simulink model "HevP4ReferenceApplication"  (R2020a)
settings: Solver=ode23tb  StartTime=0  StopTime=1800  RelTol=1e-3  EnableMultiTasking=on
undefined symbols (not defined in the file): sigbuilder_block
libraries: autolibshared x2
(part 2 of 2)

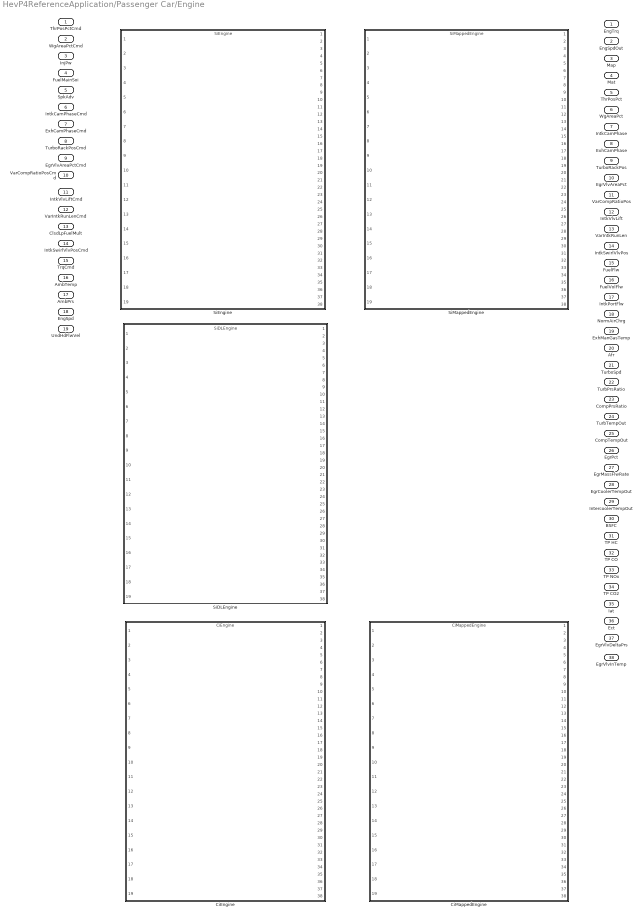
== system HevP4ReferenceApplication/Passenger Car/Engine ==
  ThrPosPctCmd : Inport
  WgAreaPctCmd : Inport  Port=2
  InjPw : Inport  Port=3
  FuelMainSoi : Inport  Port=4
  SpkAdv : Inport  Port=5
  IntkCamPhaseCmd : Inport  Port=6
  ExhCamPhaseCmd : Inport  Port=7
  TurboRackPosCmd : Inport  Port=8
  EgrVlvAreaPctCmd : Inport  Port=9
  VarCompRatioPosCmd : Inport  Port=10
  IntkVlvLiftCmd : Inport  Port=11
  VarIntkRunLenCmd : Inport  Port=12
  ClsdLpFuelMult : Inport  Port=13
  IntkSwirlVlvPosCmd : Inport  Port=14
  TrqCmd : Inport  Port=15
  AmbTemp : Inport  Port=16
  AmbPrs : Inport  Port=17
  EngSpd : Inport  Port=18
  UndHdFlwVel : Inport  Port=19
  CiEngine : ModelReference  ModelNameDialog=CiEngine.slx  SimulationMode=Normal  VariantControl=CiEngine  ModelReferenceVersion=1.370
  CiMappedEngine : ModelReference  ModelNameDialog=CiMappedEngine.slx  SimulationMode=Normal  VariantControl=CiMappedEngine  ModelReferenceVersion=1.321
  SiDLEngine : ModelReference  ModelNameDialog=SiDLEngine  SimulationMode=Normal  VariantControl=SiDLEngine  ModelReferenceVersion=1.459
  SiEngine : ModelReference  ModelNameDialog=SiEngine.slx  SimulationMode=Normal  VariantControl=SiEngine  ModelReferenceVersion=1.573
  SiMappedEngine : ModelReference  ModelNameDialog=SiMappedEngine.slx  SimulationMode=Normal  VariantControl=SiMappedEngine  ModelReferenceVersion=1.331
  EngTrq : Outport  VectorParamsAs1DForOutWhenUnconnected=off
  EngSpdOut : Outport  Port=2  VectorParamsAs1DForOutWhenUnconnected=off
  Map : Outport  Port=3  VectorParamsAs1DForOutWhenUnconnected=off
  Mat : Outport  Port=4  VectorParamsAs1DForOutWhenUnconnected=off
  ThrPosPct : Outport  Port=5  VectorParamsAs1DForOutWhenUnconnected=off
  WgAreaPct : Outport  Port=6  VectorParamsAs1DForOutWhenUnconnected=off
  IntkCamPhase : Outport  Port=7  VectorParamsAs1DForOutWhenUnconnected=off
  ExhCamPhase : Outport  Port=8  VectorParamsAs1DForOutWhenUnconnected=off
  TurboRackPos : Outport  Port=9  VectorParamsAs1DForOutWhenUnconnected=off
  EgrVlvAreaPct : Outport  Port=10  VectorParamsAs1DForOutWhenUnconnected=off
  VarCompRatioPos : Outport  Port=11  VectorParamsAs1DForOutWhenUnconnected=off
  IntkVlvLift : Outport  Port=12  VectorParamsAs1DForOutWhenUnconnected=off
  VarIntkRunLen : Outport  Port=13  VectorParamsAs1DForOutWhenUnconnected=off
  IntkSwirlVlvPos : Outport  Port=14  VectorParamsAs1DForOutWhenUnconnected=off
  FuelFlw : Outport  Port=15  VectorParamsAs1DForOutWhenUnconnected=off
  FuelVolFlw : Outport  Port=16  VectorParamsAs1DForOutWhenUnconnected=off
  IntkPortFlw : Outport  Port=17  VectorParamsAs1DForOutWhenUnconnected=off
  NormAirChrg : Outport  Port=18  VectorParamsAs1DForOutWhenUnconnected=off
  ExhManGasTemp : Outport  Port=19  VectorParamsAs1DForOutWhenUnconnected=off
  Afr : Outport  Port=20  VectorParamsAs1DForOutWhenUnconnected=off
  TurboSpd : Outport  Port=21  VectorParamsAs1DForOutWhenUnconnected=off
  TurbPrsRatio : Outport  Port=22  VectorParamsAs1DForOutWhenUnconnected=off
  CompPrsRatio : Outport  Port=23  VectorParamsAs1DForOutWhenUnconnected=off
  TurbTempOut : Outport  Port=24  VectorParamsAs1DForOutWhenUnconnected=off
  CompTempOut : Outport  Port=25  VectorParamsAs1DForOutWhenUnconnected=off
  EgrPct : Outport  Port=26  VectorParamsAs1DForOutWhenUnconnected=off
  EgrMassFlwRate : Outport  Port=27  VectorParamsAs1DForOutWhenUnconnected=off
  EgrCoolerTempOut : Outport  Port=28  VectorParamsAs1DForOutWhenUnconnected=off
  IntercoolerTempOut : Outport  Port=29  VectorParamsAs1DForOutWhenUnconnected=off
  BSFC : Outport  Port=30  VectorParamsAs1DForOutWhenUnconnected=off
  TP HC : Outport  Port=31  VectorParamsAs1DForOutWhenUnconnected=off
  TP CO : Outport  Port=32  VectorParamsAs1DForOutWhenUnconnected=off
  TP NOx : Outport  Port=33  VectorParamsAs1DForOutWhenUnconnected=off
  TP CO2 : Outport  Port=34  VectorParamsAs1DForOutWhenUnconnected=off
  Iat : Outport  Port=35  VectorParamsAs1DForOutWhenUnconnected=off
  Ect : Outport  Port=36  VectorParamsAs1DForOutWhenUnconnected=off
  EgrVlvDeltaPrs : Outport  Port=37  VectorParamsAs1DForOutWhenUnconnected=off
  EgrVlvInTemp : Outport  Port=38  VectorParamsAs1DForOutWhenUnconnected=off

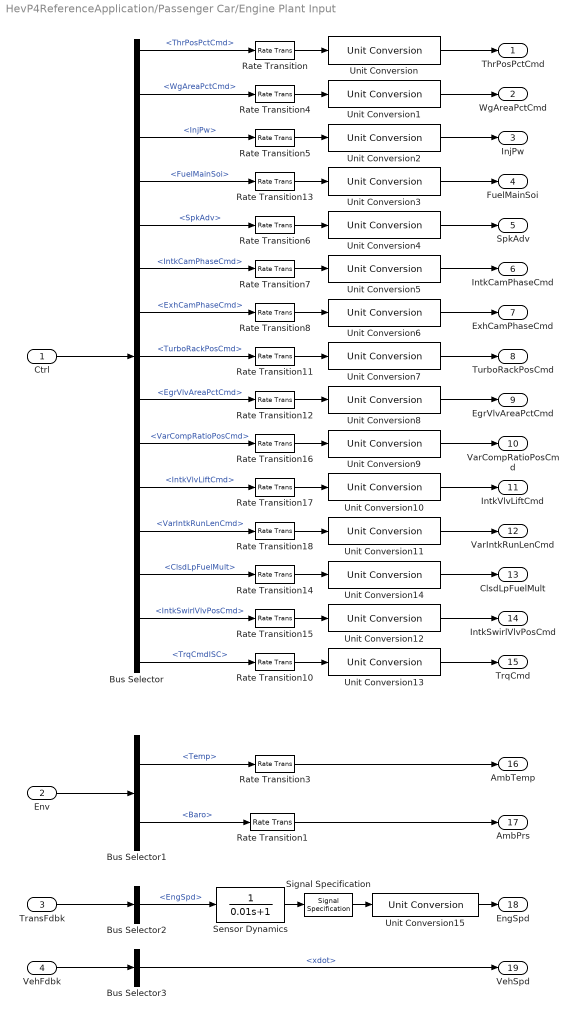
== system HevP4ReferenceApplication/Passenger Car/Engine Plant Input ==
  Ctrl : Inport
  Env : Inport  Port=2
  TransFdbk : Inport  Port=3
  VehFdbk : Inport  Port=4
  Bus Selector : BusSelector  OutputSignals=EngCtrl.ThrPosPctCmd,EngCtrl.WgAreaPctCmd,EngCtrl.InjPw,EngCtrl.FuelMainSoi,EngCtrl.SpkAdv,EngCtrl.IntkCamPhaseCmd,EngCtrl.ExhCamPhaseCmd,EngCtrl.TurboRackPosCmd,EngCtrl.EgrVlvAreaPctCmd,EngCtrl.VarCompRatioPosCmd,EngCtrl.IntkVlvLiftCmd,EngCtrl.VarIntkRunLenCmd,EngCtrl.ClsdLpFuelMult,EngCtrl.IntkSwirlVlvPosCmd,EngCtrl.TrqCmdISC
  Bus Selector1 : BusSelector  OutputSignals=Temp,Baro
  Bus Selector2 : BusSelector  OutputSignals=EngSpd
  Bus Selector3 : BusSelector  OutputSignals=xdot
  Rate Transition{,1,3..8,10..18} (17 alike) : RateTransition  Deterministic=off
  Sensor Dynamics : TransferFcn  Denominator=[0.01 1]
  Signal Specification : SignalSpecification  Unit=rad/s
  Unit Conversion{,1..15} (16 alike) : UnitConversion
  ThrPosPctCmd : Outport  VectorParamsAs1DForOutWhenUnconnected=off
  WgAreaPctCmd : Outport  Port=2  VectorParamsAs1DForOutWhenUnconnected=off
  InjPw : Outport  Port=3  VectorParamsAs1DForOutWhenUnconnected=off
  FuelMainSoi : Outport  Port=4  VectorParamsAs1DForOutWhenUnconnected=off
  SpkAdv : Outport  Port=5  VectorParamsAs1DForOutWhenUnconnected=off
  IntkCamPhaseCmd : Outport  Port=6  VectorParamsAs1DForOutWhenUnconnected=off
  ExhCamPhaseCmd : Outport  Port=7  VectorParamsAs1DForOutWhenUnconnected=off
  TurboRackPosCmd : Outport  Port=8  VectorParamsAs1DForOutWhenUnconnected=off
  EgrVlvAreaPctCmd : Outport  Port=9  VectorParamsAs1DForOutWhenUnconnected=off
  VarCompRatioPosCmd : Outport  Port=10  VectorParamsAs1DForOutWhenUnconnected=off
  IntkVlvLiftCmd : Outport  Port=11  VectorParamsAs1DForOutWhenUnconnected=off
  VarIntkRunLenCmd : Outport  Port=12  VectorParamsAs1DForOutWhenUnconnected=off
  ClsdLpFuelMult : Outport  Port=13  VectorParamsAs1DForOutWhenUnconnected=off
  IntkSwirlVlvPosCmd : Outport  Port=14  VectorParamsAs1DForOutWhenUnconnected=off
  TrqCmd : Outport  Port=15  VectorParamsAs1DForOutWhenUnconnected=off
  AmbTemp : Outport  Port=16  VectorParamsAs1DForOutWhenUnconnected=off
  AmbPrs : Outport  Port=17  VectorParamsAs1DForOutWhenUnconnected=off
  EngSpd : Outport  Port=18  VectorParamsAs1DForOutWhenUnconnected=off
  VehSpd : Outport  Port=19  VectorParamsAs1DForOutWhenUnconnected=off
  wires:
  Env/1 -> Bus Selector1/1
  Bus Selector1/2 -> Rate Transition1/1  "<Baro>"
  Rate Transition1/1 -> AmbPrs/1
  TransFdbk/1 -> Bus Selector2/1
  Bus Selector2/1 -> Sensor Dynamics/1  "<EngSpd>"
  Rate Transition3/1 -> AmbTemp/1
  Bus Selector1/1 -> Rate Transition3/1  "<Temp>"
  VehFdbk/1 -> Bus Selector3/1
  Bus Selector3/1 -> VehSpd/1  "<xdot>"
  Sensor Dynamics/1 -> Signal Specification/1
  Ctrl/1 -> Bus Selector/1
  Rate Transition15/1 -> Unit Conversion12/1
  Rate Transition14/1 -> Unit Conversion14/1
  Rate Transition18/1 -> Unit Conversion11/1
  Rate Transition17/1 -> Unit Conversion10/1
  Rate Transition16/1 -> Unit Conversion9/1
  Rate Transition13/1 -> Unit Conversion3/1
  Rate Transition/1 -> Unit Conversion/1
  Rate Transition4/1 -> Unit Conversion1/1
  Rate Transition5/1 -> Unit Conversion2/1
  Rate Transition6/1 -> Unit Conversion4/1
  Rate Transition7/1 -> Unit Conversion5/1
  Rate Transition8/1 -> Unit Conversion6/1
  Rate Transition10/1 -> Unit Conversion13/1
  Rate Transition11/1 -> Unit Conversion7/1
  Rate Transition12/1 -> Unit Conversion8/1
  Bus Selector/1 -> Rate Transition/1  "<ThrPosPctCmd>"
  Bus Selector/2 -> Rate Transition4/1  "<WgAreaPctCmd>"
  Bus Selector/3 -> Rate Transition5/1  "<InjPw>"
  Bus Selector/4 -> Rate Transition13/1  "<FuelMainSoi>"
  Bus Selector/5 -> Rate Transition6/1  "<SpkAdv>"
  Bus Selector/6 -> Rate Transition7/1  "<IntkCamPhaseCmd>"
  Bus Selector/7 -> Rate Transition8/1  "<ExhCamPhaseCmd>"
  Bus Selector/8 -> Rate Transition11/1  "<TurboRackPosCmd>"
  Bus Selector/9 -> Rate Transition12/1  "<EgrVlvAreaPctCmd>"
  Bus Selector/10 -> Rate Transition16/1  "<VarCompRatioPosCmd>"
  Bus Selector/11 -> Rate Transition17/1  "<IntkVlvLiftCmd>"
  Bus Selector/12 -> Rate Transition18/1  "<VarIntkRunLenCmd>"
  Bus Selector/13 -> Rate Transition14/1  "<ClsdLpFuelMult>"
  Bus Selector/14 -> Rate Transition15/1  "<IntkSwirlVlvPosCmd>"
  Bus Selector/15 -> Rate Transition10/1  "<TrqCmdISC>"
  Unit Conversion11/1 -> VarIntkRunLenCmd/1
  Unit Conversion8/1 -> EgrVlvAreaPctCmd/1
  Unit Conversion12/1 -> IntkSwirlVlvPosCmd/1
  Unit Conversion14/1 -> ClsdLpFuelMult/1
  Unit Conversion/1 -> ThrPosPctCmd/1
  Unit Conversion1/1 -> WgAreaPctCmd/1
  Unit Conversion3/1 -> FuelMainSoi/1
  Unit Conversion2/1 -> InjPw/1
  Unit Conversion9/1 -> VarCompRatioPosCmd/1
  Unit Conversion4/1 -> SpkAdv/1
  Unit Conversion7/1 -> TurboRackPosCmd/1
  Unit Conversion13/1 -> TrqCmd/1
  Unit Conversion10/1 -> IntkVlvLiftCmd/1
  Unit Conversion6/1 -> ExhCamPhaseCmd/1
  Unit Conversion5/1 -> IntkCamPhaseCmd/1
  Unit Conversion15/1 -> EngSpd/1
  Signal Specification/1 -> Unit Conversion15/1

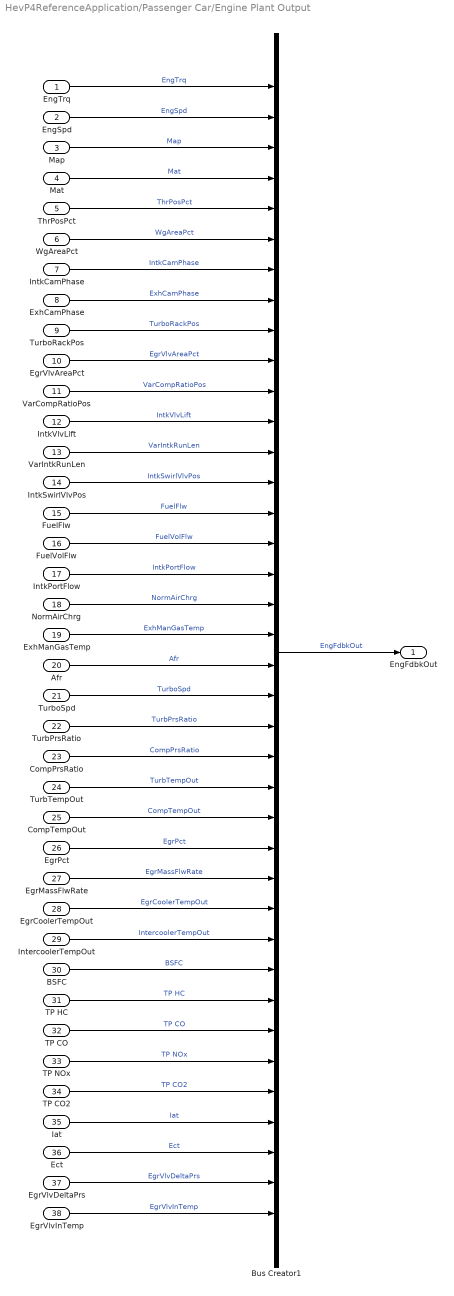
== system HevP4ReferenceApplication/Passenger Car/Engine Plant Output ==
  EngTrq : Inport
  EngSpd : Inport  Port=2
  Map : Inport  Port=3
  Mat : Inport  Port=4
  ThrPosPct : Inport  Port=5
  WgAreaPct : Inport  Port=6
  IntkCamPhase : Inport  Port=7
  ExhCamPhase : Inport  Port=8
  TurboRackPos : Inport  Port=9
  EgrVlvAreaPct : Inport  Port=10
  VarCompRatioPos : Inport  Port=11
  IntkVlvLift : Inport  Port=12
  VarIntkRunLen : Inport  Port=13
  IntkSwirlVlvPos : Inport  Port=14
  FuelFlw : Inport  Port=15
  FuelVolFlw : Inport  Port=16
  IntkPortFlow : Inport  Port=17
  NormAirChrg : Inport  Port=18
  ExhManGasTemp : Inport  Port=19
  Afr : Inport  Port=20
  TurboSpd : Inport  Port=21
  TurbPrsRatio : Inport  Port=22
  CompPrsRatio : Inport  Port=23
  TurbTempOut : Inport  Port=24
  CompTempOut : Inport  Port=25
  EgrPct : Inport  Port=26
  EgrMassFlwRate : Inport  Port=27
  EgrCoolerTempOut : Inport  Port=28
  IntercoolerTempOut : Inport  Port=29
  BSFC : Inport  Port=30
  TP HC : Inport  Port=31
  TP CO : Inport  Port=32
  TP NOx : Inport  Port=33
  TP CO2 : Inport  Port=34
  Iat : Inport  Port=35
  Ect : Inport  Port=36
  EgrVlvDeltaPrs : Inport  Port=37
  EgrVlvInTemp : Inport  Port=38
  Bus Creator1 : BusCreator  Inputs=38
  EngFdbkOut : Outport  VectorParamsAs1DForOutWhenUnconnected=off
  wires:
  VarIntkRunLen/1 -> Bus Creator1/13  "VarIntkRunLen"
  IntkVlvLift/1 -> Bus Creator1/12  "IntkVlvLift"
  VarCompRatioPos/1 -> Bus Creator1/11  "VarCompRatioPos"
  WgAreaPct/1 -> Bus Creator1/6  "WgAreaPct"
  TurboRackPos/1 -> Bus Creator1/9  "TurboRackPos"
  ThrPosPct/1 -> Bus Creator1/5  "ThrPosPct"
  EngTrq/1 -> Bus Creator1/1  "EngTrq"
  Mat/1 -> Bus Creator1/4  "Mat"
  Map/1 -> Bus Creator1/3  "Map"
  EngSpd/1 -> Bus Creator1/2  "EngSpd"
  IntkCamPhase/1 -> Bus Creator1/7  "IntkCamPhase"
  ExhCamPhase/1 -> Bus Creator1/8  "ExhCamPhase"
  EgrVlvAreaPct/1 -> Bus Creator1/10  "EgrVlvAreaPct"
  Bus Creator1/1 -> EngFdbkOut/1  "EngFdbkOut"
  IntkSwirlVlvPos/1 -> Bus Creator1/14  "IntkSwirlVlvPos"
  FuelFlw/1 -> Bus Creator1/15  "FuelFlw"
  FuelVolFlw/1 -> Bus Creator1/16  "FuelVolFlw"
  IntkPortFlow/1 -> Bus Creator1/17  "IntkPortFlow"
  NormAirChrg/1 -> Bus Creator1/18  "NormAirChrg"
  ExhManGasTemp/1 -> Bus Creator1/19  "ExhManGasTemp"
  Afr/1 -> Bus Creator1/20  "Afr"
  TurboSpd/1 -> Bus Creator1/21  "TurboSpd"
  TurbPrsRatio/1 -> Bus Creator1/22  "TurbPrsRatio"
  CompPrsRatio/1 -> Bus Creator1/23  "CompPrsRatio"
  TurbTempOut/1 -> Bus Creator1/24  "TurbTempOut"
  CompTempOut/1 -> Bus Creator1/25  "CompTempOut"
  EgrPct/1 -> Bus Creator1/26  "EgrPct"
  EgrMassFlwRate/1 -> Bus Creator1/27  "EgrMassFlwRate"
  EgrCoolerTempOut/1 -> Bus Creator1/28  "EgrCoolerTempOut"
  IntercoolerTempOut/1 -> Bus Creator1/29  "IntercoolerTempOut"
  BSFC/1 -> Bus Creator1/30  "BSFC"
  TP HC/1 -> Bus Creator1/31  "TP HC"
  TP CO/1 -> Bus Creator1/32  "TP CO"
  TP NOx/1 -> Bus Creator1/33  "TP NOx"
  TP CO2/1 -> Bus Creator1/34  "TP CO2"
  Iat/1 -> Bus Creator1/35  "Iat"
  Ect/1 -> Bus Creator1/36  "Ect"
  EgrVlvDeltaPrs/1 -> Bus Creator1/37  "EgrVlvDeltaPrs"
  EgrVlvInTemp/1 -> Bus Creator1/38  "EgrVlvInTemp"

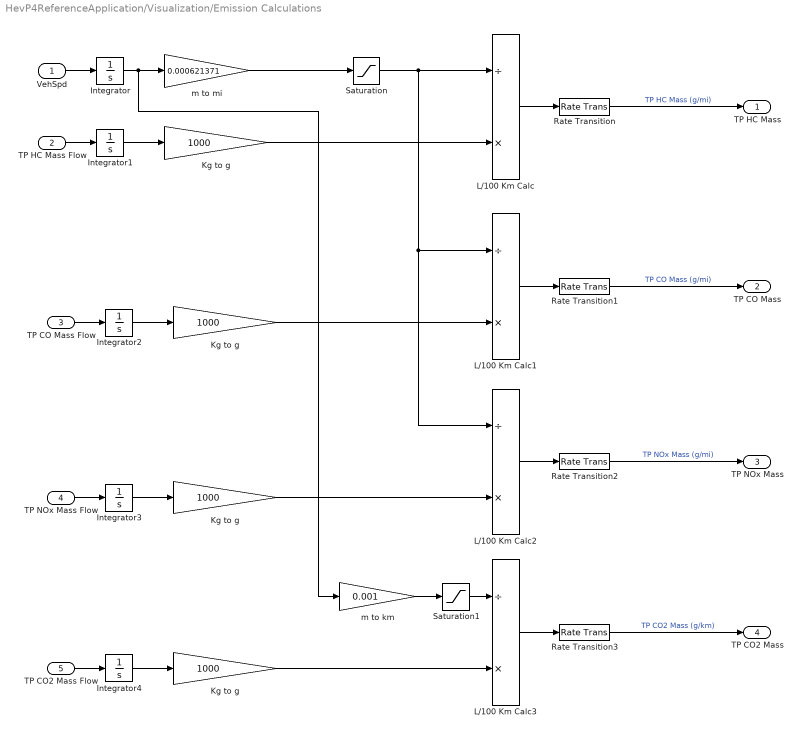
== system HevP4ReferenceApplication/Visualization/Emission Calculations ==
  VehSpd : Inport
  TP HC Mass Flow : Inport  Port=2
  TP CO Mass Flow : Inport  Port=3
  TP NOx Mass Flow : Inport  Port=4
  TP CO2 Mass Flow : Inport  Port=5
  Integrator{,1..4} (5 alike) : Integrator
  Kg to g : Gain  Gain=1000
  "Kg to g " : Gain  Gain=1000
  "Kg to g  " : Gain  Gain=1000
  "Kg to g   " : Gain  Gain=1000
  L/100 Km Calc{,1..3} (4 alike) : Product  Inputs=/*
  Rate Transition{,1..3} (4 alike) : RateTransition  Deterministic=off
  Saturation : Saturate  UpperLimit=Inf  LowerLimit=0.2
  Saturation1 : Saturate  UpperLimit=Inf  LowerLimit=1
  m to km : Gain  Gain=0.001
  m to mi : Gain  Gain=0.000621371
  TP HC Mass : Outport  VectorParamsAs1DForOutWhenUnconnected=off
  TP CO Mass : Outport  Port=2  VectorParamsAs1DForOutWhenUnconnected=off
  TP NOx Mass : Outport  Port=3  VectorParamsAs1DForOutWhenUnconnected=off
  TP CO2 Mass : Outport  Port=4  VectorParamsAs1DForOutWhenUnconnected=off
  wires:
  L/100 Km Calc/1 -> Rate Transition/1
  VehSpd/1 -> Integrator/1
  m to mi/1 -> Saturation/1
  Saturation/1 -> L/100 Km Calc2/1, L/100 Km Calc1/1, L/100 Km Calc/1
  TP HC Mass Flow/1 -> Integrator1/1
  Integrator1/1 -> Kg to g/1
  Integrator/1 -> m to km/1, m to mi/1
  Kg to g/1 -> L/100 Km Calc/2
  TP CO Mass Flow/1 -> Integrator2/1
  Integrator2/1 -> "Kg to g "/1
  "Kg to g "/1 -> L/100 Km Calc1/2
  TP NOx Mass Flow/1 -> Integrator3/1
  Integrator3/1 -> "Kg to g  "/1
  "Kg to g  "/1 -> L/100 Km Calc2/2
  L/100 Km Calc1/1 -> Rate Transition1/1
  L/100 Km Calc2/1 -> Rate Transition2/1
  TP CO2 Mass Flow/1 -> Integrator4/1
  Integrator4/1 -> "Kg to g   "/1
  "Kg to g   "/1 -> L/100 Km Calc3/2
  L/100 Km Calc3/1 -> Rate Transition3/1
  Saturation1/1 -> L/100 Km Calc3/1
  m to km/1 -> Saturation1/1
  Rate Transition/1 -> TP HC Mass/1  "TP HC Mass (g/mi)"
  Rate Transition1/1 -> TP CO Mass/1  "TP CO Mass (g/mi)"
  Rate Transition2/1 -> TP NOx Mass/1  "TP NOx Mass (g/mi)"
  Rate Transition3/1 -> TP CO2 Mass/1  "TP CO2 Mass (g/km)"

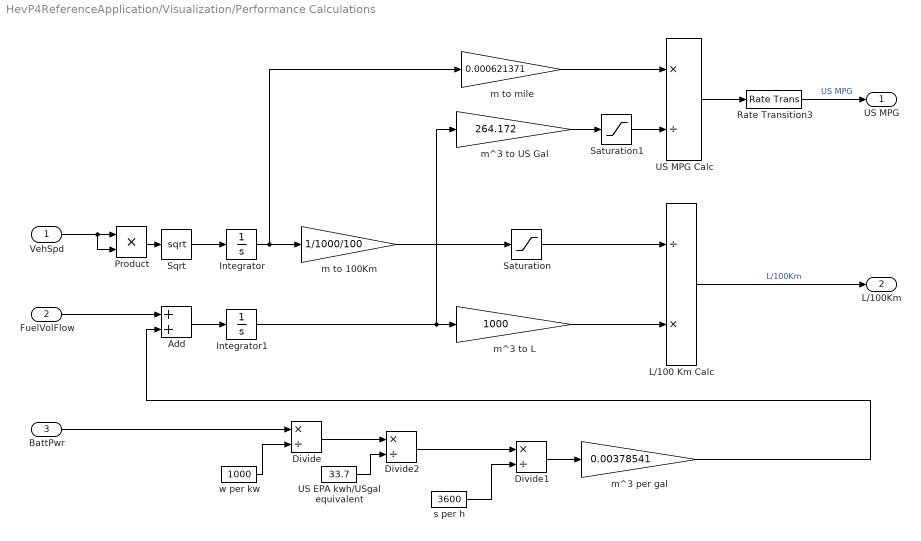
== system HevP4ReferenceApplication/Visualization/Performance Calculations ==
  VehSpd : Inport
  FuelVolFlow : Inport  Port=2
  BattPwr : Inport  Port=3
  Add : Sum
  Divide : Product  Inputs=*/
  Divide1 : Product  Inputs=*/
  Divide2 : Product  Inputs=*/
  Integrator : Integrator
  Integrator1 : Integrator
  L/100 Km Calc : Product  Inputs=/*
  Product : Product
  Rate Transition3 : RateTransition  Deterministic=off
  Saturation : Saturate  UpperLimit=Inf  LowerLimit=0.001
  Saturation1 : Saturate  UpperLimit=Inf  LowerLimit=1e-3
  Sqrt : Sqrt  SaturateOnIntegerOverflow=on
  US EPA kwh/USgal equivalent : Constant  Value=33.7
  US MPG Calc : Product  Inputs=*/
  m to 100Km : Gain  Gain=1/1000/100
  m to mile : Gain  Gain=0.000621371
  m^3 per gal : Gain  Gain=0.00378541
  m^3 to L : Gain  Gain=1000
  m^3 to US Gal : Gain  Gain=264.172
  s per h : Constant  Value=3600
  w per kw : Constant  Value=1000
  US MPG : Outport  VectorParamsAs1DForOutWhenUnconnected=off
  L/100Km : Outport  Port=2  VectorParamsAs1DForOutWhenUnconnected=off
  wires:
  m^3 to US Gal/1 -> Saturation1/1
  m^3 to L/1 -> L/100 Km Calc/2
  Integrator/1 -> m to mile/1, m to 100Km/1
  m to mile/1 -> US MPG Calc/1
  FuelVolFlow/1 -> Add/1
  Integrator1/1 -> m^3 to US Gal/1, m^3 to L/1
  Saturation/1 -> L/100 Km Calc/1
  m to 100Km/1 -> Saturation/1
  L/100 Km Calc/1 -> L/100Km/1  "L/100Km"
  US MPG Calc/1 -> Rate Transition3/1
  Saturation1/1 -> US MPG Calc/2
  Rate Transition3/1 -> US MPG/1  "US MPG"
  w per kw/1 -> Divide/2
  Divide/1 -> Divide2/1
  Divide2/1 -> Divide1/1
  s per h/1 -> Divide1/2
  Divide1/1 -> m^3 per gal/1
  Add/1 -> Integrator1/1
  m^3 per gal/1 -> Add/2
  US EPA kwh/USgal equivalent/1 -> Divide2/2
  BattPwr/1 -> Divide/1
  Sqrt/1 -> Integrator/1
  Product/1 -> Sqrt/1
  VehSpd/1 -> Product/2, Product/1

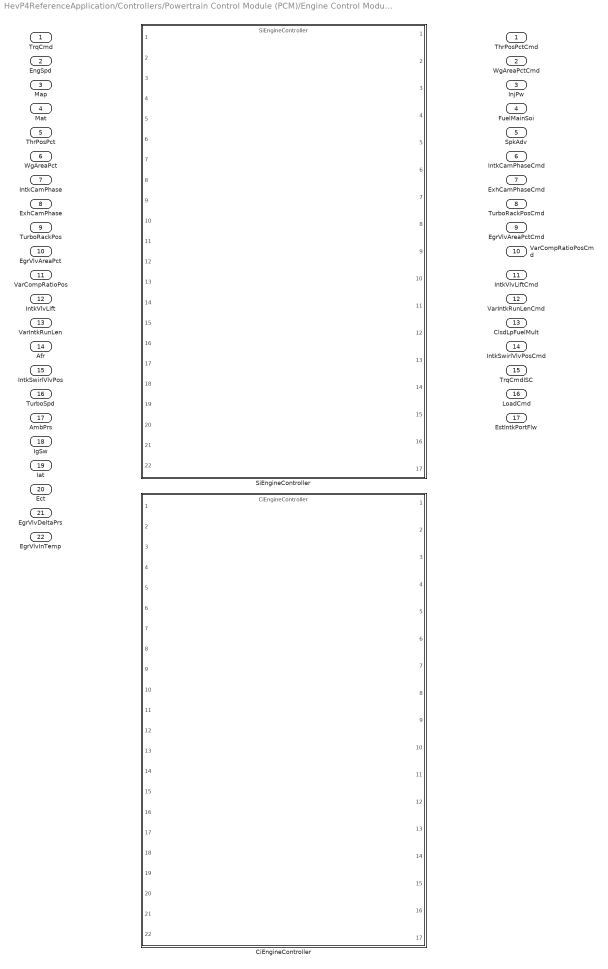
== system HevP4ReferenceApplication/Controllers/Powertrain Control Module (PCM)/Engine Control Module (ECM) ==
  TrqCmd : Inport
  EngSpd : Inport  Port=2
  Map : Inport  Port=3
  Mat : Inport  Port=4
  ThrPosPct : Inport  Port=5
  WgAreaPct : Inport  Port=6
  IntkCamPhase : Inport  Port=7
  ExhCamPhase : Inport  Port=8
  TurboRackPos : Inport  Port=9
  EgrVlvAreaPct : Inport  Port=10
  VarCompRatioPos : Inport  Port=11
  IntkVlvLift : Inport  Port=12
  VarIntkRunLen : Inport  Port=13
  Afr : Inport  Port=14
  IntkSwirlVlvPos : Inport  Port=15
  TurboSpd : Inport  Port=16
  AmbPrs : Inport  Port=17
  IgSw : Inport  Port=18
  Iat : Inport  Port=19
  Ect : Inport  Port=20
  EgrVlvDeltaPrs : Inport  Port=21
  EgrVlvInTemp : Inport  Port=22
  CiEngineController : ModelReference  ModelNameDialog=CiEngineController.slx  SimulationMode=Normal  VariantControl=CiEngineController  ModelReferenceVersion=1.243
  SiEngineController : ModelReference  ModelNameDialog=SiEngineController.slx  SimulationMode=Normal  VariantControl=SiEngineController  ModelReferenceVersion=1.306
  ThrPosPctCmd : Outport  VectorParamsAs1DForOutWhenUnconnected=off
  WgAreaPctCmd : Outport  Port=2  VectorParamsAs1DForOutWhenUnconnected=off
  InjPw : Outport  Port=3  VectorParamsAs1DForOutWhenUnconnected=off
  FuelMainSoi : Outport  Port=4  VectorParamsAs1DForOutWhenUnconnected=off
  SpkAdv : Outport  Port=5  VectorParamsAs1DForOutWhenUnconnected=off
  IntkCamPhaseCmd : Outport  Port=6  VectorParamsAs1DForOutWhenUnconnected=off
  ExhCamPhaseCmd : Outport  Port=7  VectorParamsAs1DForOutWhenUnconnected=off
  TurboRackPosCmd : Outport  Port=8  VectorParamsAs1DForOutWhenUnconnected=off
  EgrVlvAreaPctCmd : Outport  Port=9  VectorParamsAs1DForOutWhenUnconnected=off
  VarCompRatioPosCmd : Outport  Port=10  VectorParamsAs1DForOutWhenUnconnected=off
  IntkVlvLiftCmd : Outport  Port=11  VectorParamsAs1DForOutWhenUnconnected=off
  VarIntkRunLenCmd : Outport  Port=12  VectorParamsAs1DForOutWhenUnconnected=off
  ClsdLpFuelMult : Outport  Port=13  VectorParamsAs1DForOutWhenUnconnected=off
  IntkSwirlVlvPosCmd : Outport  Port=14  VectorParamsAs1DForOutWhenUnconnected=off
  TrqCmdISC : Outport  Port=15  VectorParamsAs1DForOutWhenUnconnected=off
  LoadCmd : Outport  Port=16  VectorParamsAs1DForOutWhenUnconnected=off
  EstIntkPortFlw : Outport  Port=17  VectorParamsAs1DForOutWhenUnconnected=off

== system HevP4ReferenceApplication/Controllers/Powertrain Control Module (PCM)/Hybrid Control Module (HCM) ==
  "AccelPdl " : Inport
  "DecelPdl " : Inport  Port=2
  "VehSpdFdbk " : Inport  Port=3
  "EngSpdFdbk " : Inport  Port=4
  "BattSoc " : Inport  Port=5
  "BattPwr " : Inport  Port=6
  "MotSpd " : Inport  Port=7
  "EngTrqOut " : Inport  Port=8
  "Cltch1State " : Inport  Port=9
  "Cltch2State " : Inport  Port=10
  "Chrg " : Inport  Port=11
  "BattV " : Inport  Port=12
  "TransGear " : Inport  Port=13
  Hybrid Control Module (HCM) - Optimal : ModelReference  ModelNameDialog=HevP4OptimalController  SimulationMode=Normal  VariantControl=4  ModelReferenceVersion=1.3995
  " EngTrqCmd" : Outport  VectorParamsAs1DForOutWhenUnconnected=off
  " MotTrqCmd" : Outport  Port=2  VectorParamsAs1DForOutWhenUnconnected=off
  " BrkCmd" : Outport  Port=3  VectorParamsAs1DForOutWhenUnconnected=off
  " Cltch1Cmd" : Outport  Port=4  VectorParamsAs1DForOutWhenUnconnected=off
  " StartCmd" : Outport  Port=5  VectorParamsAs1DForOutWhenUnconnected=off
  " Neutral" : Outport  Port=6  VectorParamsAs1DForOutWhenUnconnected=off
  " WhlTrqCmd" : Outport  Port=7  VectorParamsAs1DForOutWhenUnconnected=off

== system HevP4ReferenceApplication/Longitudinal Driver/Closed Loop/Ignition Switch Profile1 ==
  Demux : Demux  Tag=STV Demux  Outputs=1
      settings: DisplayOption=none
  FromWs : FromWorkspace  Tag=STV FromWs  VariableName=tuvar
      SigBuilderData=|
      | common.afterFinalStr = 'Extrapolate'
      | common.sampleTime = 0
      | dataSet.timeRange = [0 10]
      | dataSet.name = 'Group 1'
      | sbobj.Groups.Name = 'Group 1'
      | sbobj.Groups.Signals.Name = 'IGSW'
      | sbobj.Groups.Signals.XData = [0 5 5 6 6 10]
      | sbobj.Groups.Signals.YData = [0 0 1 1 0 0]
  IGSW : Outport  Tag=STV Outport  VectorParamsAs1DForOutWhenUnconnected=off
  wires:
  Demux/1 -> IGSW/1
  FromWs/1 -> Demux/1

== system HevP4ReferenceApplication/Longitudinal Driver/Closed Loop/Optional Stationary Charging ==
  note: Setup for FTP75, allow charging
      | between 1490-1860 secs when
      | vehicle is stopped
  Charge Profile : Subsystem  Tag=STV Subsys  LoadFcn=sigbuilder_block('load');  StartFcn=sigbuilder_block('start');  StopFcn=sigbuilder_block('stop');  ClipboardFcn=sigbuilder_block('clipboard');  mask(Sigbuilder block){tuvar=[0:10]}
      mask help: Simulink:masks:SigbuilderBlock_MD
      mask init:
      | if ~strcmp(get_param(bdroot(gcbh),'SimulationStatus'),'stopped') tuvar = sigbuilder_block('maskInit'); end
      settings: CopyFcn=sigbuilder_block('copy');  DeleteFcn=sigbuilder_block('delete');  ModelCloseFcn=sigbuilder_block('modelClose');  PreSaveFcn=sigbuilder_block('preSave');  PauseFcn=sigbuilder_block('pause');  ContinueFcn=sigbuilder_block('continue');  NameChangeFcn=sigbuilder_block('namechange');  OpenFcn=sigbuilder_block('open',[6 30 1428 771.75 ]);  CloseFcn=sigbuilder_block('close');
      mask Display: plot(0, 0, 100, 100,[2, 2, 32, 32, 2], [68, 8, 8, 68, 68],[32, 2], [38, 38], [32, 19, 2],[53, 60, 44], [32, 17, 17, 2],[16, 16, 31, 31]);txt = getActiveGroup(gcbh);text(2, 100, txt,'verticalAlignment', 'top');
  Constant1 : Constant  Value=false
  Data Type Conversion1 : DataTypeConversion  OutDataTypeStr=boolean
  Manual Switch1 : ManualSwitch
  Charge : Outport  VectorParamsAs1DForOutWhenUnconnected=off
  wires:
  Manual Switch1/1 -> Charge/1  "Charge"
  Charge Profile/1(IGSW) -> Data Type Conversion1/1
  Data Type Conversion1/1 -> Manual Switch1/2
  Constant1/1 -> Manual Switch1/1

== system HevP4ReferenceApplication/Passenger Car/Electric Plant/Electric Machine ==
  MotTrqCmd : Inport
  MotSpd : Inport  Port=2
  BusVolt : Inport  Port=3
  MotMapped : ModelReference  ModelNameDialog=MotMappedP4  SimulationMode=Normal  VariantControl=1  ModelReferenceVersion=1.376
  MotTrq : Outport  VectorParamsAs1DForOutWhenUnconnected=off
  MotCurr : Outport  Port=2  VectorParamsAs1DForOutWhenUnconnected=off

== system HevP4ReferenceApplication/Longitudinal Driver/Closed Loop/Optional Stationary Charging/Charge Profile ==
  Demux : Demux  Tag=STV Demux  Outputs=1
      settings: DisplayOption=none
  FromWs : FromWorkspace  Tag=STV FromWs  VariableName=tuvar
      SigBuilderData=|
      | common.afterFinalStr = 'Extrapolate'
      | common.sampleTime = 0
      | dataSet.timeRange = [0 2474]
      | dataSet.name = 'Group 1'
      | sbobj.Groups.Name = 'Group 1'
      | sbobj.Groups.Signals.Name = 'IGSW'
      | sbobj.Groups.Signals.XData = [0 1490 1490 1860 1860 2474]
      | sbobj.Groups.Signals.YData = [0 0 1 1 0 0]
      | sbobj.Groups.TimeRange = [0 2474]
  IGSW : Outport  Tag=STV Outport  VectorParamsAs1DForOutWhenUnconnected=off
  wires:
  FromWs/1 -> Demux/1
  Demux/1 -> IGSW/1
